simulink model "simulink_Lab4"  (R2022a)
settings: Solver=FixedStepAuto  StartTime=0.0  StopTime=10.0  FixedStep=1e-3  RelTol=1e-3
values from neighbouring files (symbols this model uses):
  C = 1e-6    (= 1e-06)    [simulink_Lab4_script.m]
  R = 1e3    (= 1000)    [simulink_Lab4_script.m]
settings Model: Creator=bebawy  LastModifiedBy=bebawy

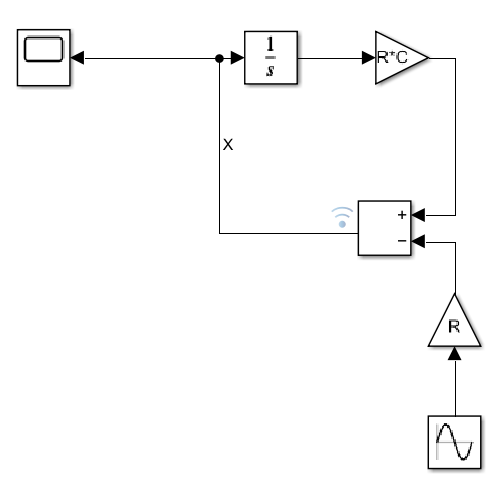
[thumbnail: Simulink's stored preview of the top-level diagram]
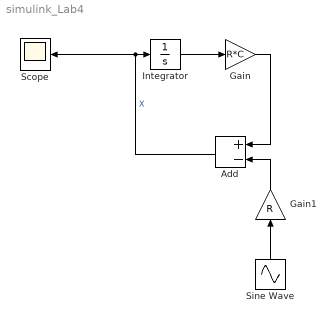
== system simulink_Lab4 ==
  Add : Sum  Inputs=+-
  Gain : Gain  Gain=R*C
  Gain1 : Gain  Gain=R
  Integrator : Integrator
  Scope : Scope
  Sine Wave : Sin  Amplitude=5  Frequency=2*pi  SampleTime=0
  wires:
  Gain/1 -> Add/1
  Sine Wave/1 -> Gain1/1
  Gain1/1 -> Add/2
  Integrator/1 -> Gain/1
  Add/1 -> Scope/1, Integrator/1  "X"
